simulink model "simulink_hw1"  (R2021a)
settings: Solver=VariableStepAuto  StartTime=0.0  StopTime=60  RelTol=1e-3
settings Model: Creator=paul8  LastModifiedBy=paul8
settings GRTTargetCC: RTWCAPISignals=on  RTWCAPIParams=on

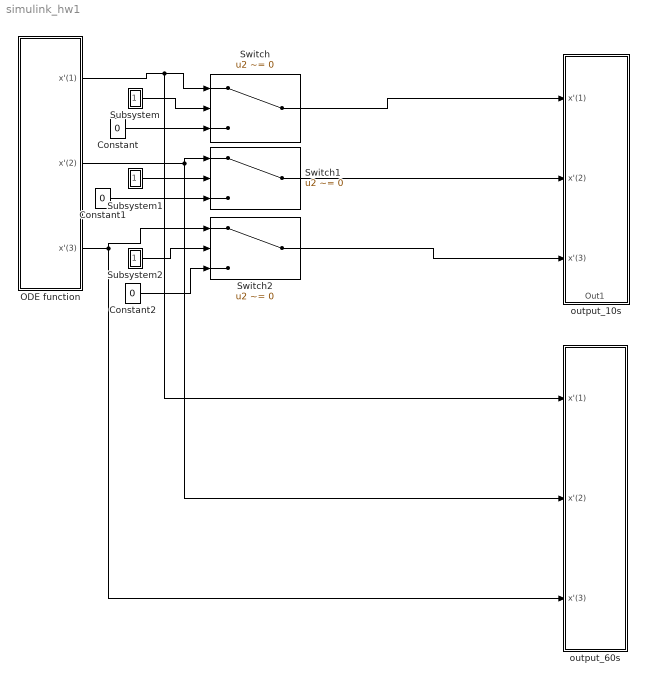
== system simulink_hw1 ==
  Constant : Constant  Value=0
  Constant1 : Constant  Value=0
  Constant2 : Constant  Value=0
  ODE function : Subsystem
  Subsystem : Subsystem
  Subsystem1 : Subsystem
  Subsystem2 : Subsystem
  Switch : Switch  Criteria=u2 ~= 0
  Switch1 : Switch  Criteria=u2 ~= 0
  Switch2 : Switch  Criteria=u2 ~= 0
  output_10s : Subsystem
      settings: PortSchema="{\"entries\":[{\"content\":{\"sides\":[{\"content\":{\"connectorIds\":[\"In1\",\"In2\",\"In3\"]},\"type\":\"ConnectorPlacement.EquallySpacedRectSide\",\"uuid\":\"c6f3c5af-19fb-40cd-a8ce-95397d139a2c\"},{\"content\":{\"connectorIds\":[],\"side\":\"RIGHT\"},\"type\":\"ConnectorPlacement.EquallySpacedRectSide\",\"uuid\":\"60b68ede-43ec-4a31-ab19-14d16abf8bcc\"},{\"content\":{\"connectorIds\":[],\"side\":\"TOP\"},\"type\":\"ConnectorPlacement.EquallySpacedRectSide\",\"uuid\":\"ed1afe09-cb60-4b47-b5bb-031a666a048a\"},{\"content\":{\"connectorIds\":[\"Out1\"],\"side\":\"BOTTOM\"},\"type\":\"ConnectorPlacement.EquallySpacedRectSide\",\"uuid\":\"2110696b-785b-458c-ba24-bc249324ac62\"}]},\"type\":\"ConnectorPlacement.EquallySpacedConnector\",\"uuid\":\"b19f2d45-dd69-4a9b-9418-a6613a161224\"}],\"packageUris\":[\"http://schema.mathworks.com/mf0/Connector/R2020b\"],\"version\":\"1.0\"}"
  output_60s : Subsystem
  wires:
  ODE function/1(x'(1)) -> output_60s/1(x'(1)), Switch/1
  Switch/1 -> output_10s/1(x'(1))
  Subsystem/1(Out1) -> Switch/2
  Constant/1 -> Switch/3
  ODE function/2(x'(2)) -> Switch1/1, output_60s/2(x'(2))
  Subsystem1/1(Out1) -> Switch1/2
  Constant1/1 -> Switch1/3
  Switch1/1 -> output_10s/2(x'(2))
  ODE function/3(x'(3)) -> Switch2/1, output_60s/3(x'(3))
  Subsystem2/1(Out1) -> Switch2/2
  Constant2/1 -> Switch2/3
  Switch2/1 -> output_10s/3(x'(3))

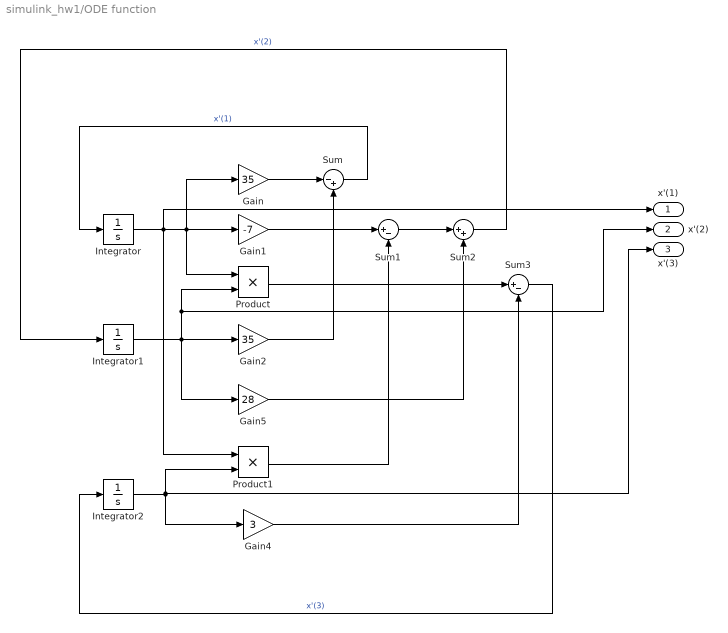
== system simulink_hw1/ODE function ==
  Gain : Gain  Gain=35
  Gain1 : Gain  Gain=-7
  Gain2 : Gain  Gain=35
  Gain4 : Gain  Gain=3
  Gain5 : Gain  Gain=28
  Integrator : Integrator  InitialCondition=-10
  Integrator1 : Integrator
  Integrator2 : Integrator  InitialCondition=37
  Product : Product
  Product1 : Product
  Sum : Sum  Inputs=|-+
  Sum1 : Sum  Inputs=|+-
  Sum2 : Sum  Inputs=|++
  Sum3 : Sum  Inputs=|+-
  x'(1) : Outport
  x'(2) : Outport  Port=2
  x'(3) : Outport  Port=3
  wires:
  Integrator2/1 -> x'(3)/1, Product1/2, Gain4/1
  Product/1 -> Sum3/1
  Gain/1 -> Sum/1
  Integrator/1 -> Product1/1, x'(1)/1, Gain/1, Product/1, Gain1/1
  Gain2/1 -> Sum/2
  Sum/1 -> Integrator/1  "x'(1)"
  Sum1/1 -> Sum2/1
  Gain4/1 -> Sum3/2
  Sum2/1 -> Integrator1/1  "x'(2)"
  Gain5/1 -> Sum2/2
  Sum3/1 -> Integrator2/1  "x'(3)"
  Integrator1/1 -> x'(2)/1, Product/2, Gain5/1, Gain2/1
  Product1/1 -> Sum1/2
  Gain1/1 -> Sum1/1

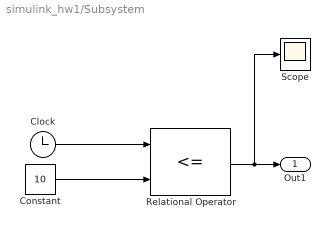
== system simulink_hw1/Subsystem ==
  Clock : Clock
      settings: Decimation=1000
  Constant : Constant  Value=10
  Relational Operator : RelationalOperator  Operator=<=  OutDataTypeStr=boolean  RndMeth=Simplest
  Scope : Scope
  Out1 : Outport
  wires:
  Clock/1 -> Relational Operator/1
  Constant/1 -> Relational Operator/2
  Relational Operator/1 -> Scope/1, Out1/1

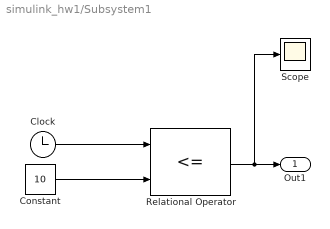
== system simulink_hw1/Subsystem1 ==
  Clock : Clock
      settings: Decimation=1000
  Constant : Constant  Value=10
  Relational Operator : RelationalOperator  Operator=<=  OutDataTypeStr=boolean  RndMeth=Simplest
  Scope : Scope
  Out1 : Outport
  wires:
  Clock/1 -> Relational Operator/1
  Constant/1 -> Relational Operator/2
  Relational Operator/1 -> Scope/1, Out1/1

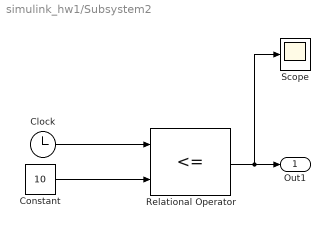
== system simulink_hw1/Subsystem2 ==
  Clock : Clock
      settings: Decimation=1000
  Constant : Constant  Value=10
  Relational Operator : RelationalOperator  Operator=<=  OutDataTypeStr=boolean  RndMeth=Simplest
  Scope : Scope
  Out1 : Outport
  wires:
  Clock/1 -> Relational Operator/1
  Constant/1 -> Relational Operator/2
  Relational Operator/1 -> Scope/1, Out1/1

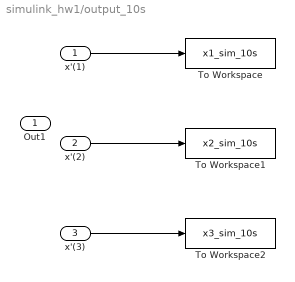
== system simulink_hw1/output_10s ==
  x'(1) : Inport
  x'(2) : Inport  Port=2
  x'(3) : Inport  Port=3
  To Workspace : ToWorkspace  VariableName=x1_sim_10s  SampleTime=0.005
  To Workspace1 : ToWorkspace  VariableName=x2_sim_10s  SampleTime=0.005
  To Workspace2 : ToWorkspace  VariableName=x3_sim_10s  SampleTime=0.005
  Out1 : Outport
  wires:
  x'(2)/1 -> To Workspace1/1
  x'(3)/1 -> To Workspace2/1
  x'(1)/1 -> To Workspace/1

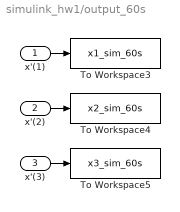
== system simulink_hw1/output_60s ==
  x'(1) : Inport
  x'(2) : Inport  Port=2
  x'(3) : Inport  Port=3
  To Workspace3 : ToWorkspace  VariableName=x1_sim_60s  SampleTime=0.005
  To Workspace4 : ToWorkspace  VariableName=x2_sim_60s  SampleTime=0.005
  To Workspace5 : ToWorkspace  VariableName=x3_sim_60s  SampleTime=0.005
  wires:
  x'(3)/1 -> To Workspace5/1
  x'(2)/1 -> To Workspace4/1
  x'(1)/1 -> To Workspace3/1
